simulink model "dng_stopwatch"  (Simulink 5.0)
settings: Solver=FixedStepDiscrete  StartTime=0.0  StopTime=inf  FixedStep=.01  RelTol=1e-3
undefined symbols (not defined in the file or in its folder): NeedleID, NeedleValue
libraries: simulink3 x1, dnglibv1 x1
settings Model: LastModifiedBy=agaltman  RTWOptions="-aEnforceIntegerDowncast=1 -aExtMode=0 -aFoldNonRolledExpr=1 -aForceParamTrailComments=0 -aGenerateComments=1 -aIgnoreCustomStorageClasses=1 -aIncHierarchyInIds=0 -aInlineInvariantSignals=0 -aLocalBlockOutputs=1 -aLogVarNameModifier=\"rt_\" -aRTWVerbose=1 -aRollThreshold=5 -aShowEliminatedStatements=1"  BooleanDataType=off

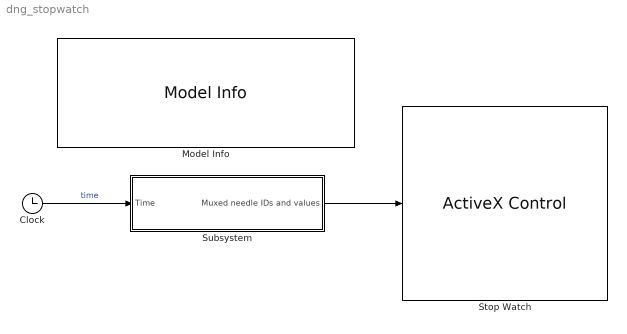
== system dng_stopwatch ==
  Clock : Clock
      settings: DisplayTime=off  Decimation=10
  Model Info : simulink3/Signals & Systems/Model Info  InitialBlockCM=none  BlockCM=none  Frame=on  DisplayStringWithTags=|  HorizontalTextAlignment=Left  LeftAlignmentValue=0.02  SourceBlockDiagram=dng_stopwatch  TagMaxNumber=20
      | This is a typical sailing stopwatch, in which
      | - The large needle spans 1 minute.
      | - The small needle on the left spans 1 second.
      | - The small needle on the right spans 15 minutes.
  Stop Watch : dnglibv1/ActiveX Control  progid=mwagauge.agaugectrl.1  connect=input  input=NeedleID,NeedleValue,NeedleID,NeedleValue,NeedleID,NeedleValue  init=hActx.configuration='Angular Gauge\Clocks\Stop Watch';  inblock=on  border=on  dialOut=0
  Subsystem : Subsystem
      settings: RTWFcnNameOpts=Auto  RTWFileNameOpts=Auto
  wires:
  Subsystem/1(Muxed needle IDs and values) -> Stop Watch/1
  Clock/1 -> Subsystem/1(Time)  "time"

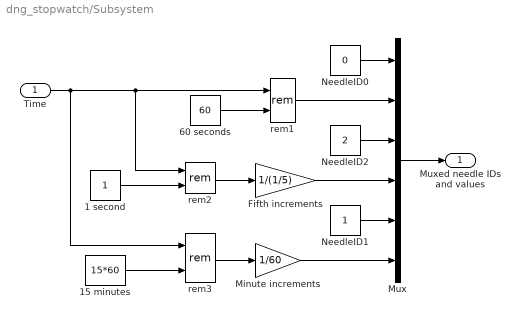
== system dng_stopwatch/Subsystem ==
  Time : Inport  Port=1  LatchInput=off
  1 second : Constant  Value=1  SettingsModeFixpt=off  OutputDataTypeScalingMode=Use data type of 'Constant value'  OutDataType=sfix(16)  OutScaling=2^0  ConRadixGroup=Use specified scaling
  15 minutes : Constant  Value=15*60  SettingsModeFixpt=off  OutputDataTypeScalingMode=Use data type of 'Constant value'  OutDataType=sfix(16)  OutScaling=2^0  ConRadixGroup=Use specified scaling
  60 seconds : Constant  Value=60  SettingsModeFixpt=off  OutputDataTypeScalingMode=Use data type of 'Constant value'  OutDataType=sfix(16)  OutScaling=2^0  ConRadixGroup=Use specified scaling
  Fifth increments : Gain  Gain=1/(1/5)  Multiplication=Element-wise(K.*u)  SaturateOnIntegerOverflow=on
  Minute increments : Gain  Gain=1/60  Multiplication=Element-wise(K.*u)  SaturateOnIntegerOverflow=on
  Mux : Mux  Inputs=6
  NeedleID0 : Constant  Value=0  SettingsModeFixpt=off  OutputDataTypeScalingMode=Use data type of 'Constant value'  OutDataType=sfix(16)  OutScaling=2^0  ConRadixGroup=Use specified scaling
  NeedleID1 : Constant  Value=1  SettingsModeFixpt=off  OutputDataTypeScalingMode=Use data type of 'Constant value'  OutDataType=sfix(16)  OutScaling=2^0  ConRadixGroup=Use specified scaling
  NeedleID2 : Constant  Value=2  SettingsModeFixpt=off  OutputDataTypeScalingMode=Use data type of 'Constant value'  OutDataType=sfix(16)  OutScaling=2^0  ConRadixGroup=Use specified scaling
  rem1 : Math  Operator=rem  OutputSignalType=auto
  rem2 : Math  Operator=rem  OutputSignalType=auto
  rem3 : Math  Operator=rem  OutputSignalType=auto
  Muxed needle IDs and values : Outport  Port=1
  wires:
  NeedleID0/1 -> Mux/1
  NeedleID2/1 -> Mux/3
  NeedleID1/1 -> Mux/5
  Fifth increments/1 -> Mux/4
  Time/1 -> rem3/1, rem2/1, rem1/1
  rem1/1 -> Mux/2
  60 seconds/1 -> rem1/2
  1 second/1 -> rem2/2
  rem2/1 -> Fifth increments/1
  Minute increments/1 -> Mux/6
  rem3/1 -> Minute increments/1
  15 minutes/1 -> rem3/2
  Mux/1 -> Muxed needle IDs and values/1
